simulink model "Assignment_2_1_compare_MIT_based_with_modified_MIT_based"  (R2023b)
settings: Solver=ode45  StartTime=0.0  StopTime=100  MaxStep=2.0  RelTol=1e-3
libraries: dspfdesign x4
settings Model: Creator=User  LastModifiedBy=User

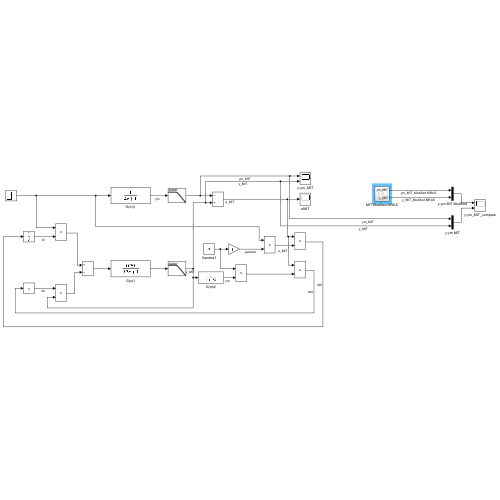
[thumbnail: Simulink's stored preview of the top-level diagram]
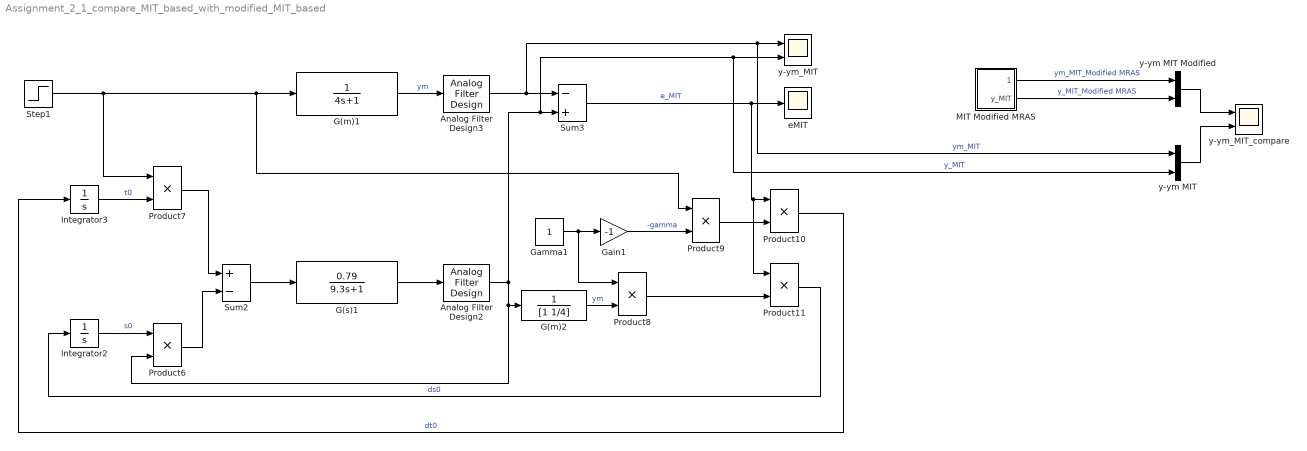
== system Assignment_2_1_compare_MIT_based_with_modified_MIT_based ==
  Analog Filter Design2 : dspfdesign/Analog Filter Design  method=Butterworth  filttype=Lowpass  N=4  Wlo=30  Whi=80  Rp=2  Rs=40
  Analog Filter Design3 : dspfdesign/Analog Filter Design  method=Butterworth  filttype=Lowpass  N=4  Wlo=30  Whi=80  Rp=2  Rs=40
  G(m)1 : TransferFcn  Denominator=[4 1]
  G(m)2 : TransferFcn  Denominator=[1 1/4]
  G(s)1 : TransferFcn  Numerator=[0.79]  Denominator=[9.3 1]
  Gain1 : Gain  Gain=-1
  Gamma1 : Constant
  Integrator2 : Integrator
  Integrator3 : Integrator
  MIT Modified MRAS : Subsystem
  Product{6..11} (6 alike) : Product
  Step1 : Step  Time=0  SampleTime=0
  Sum2 : Sum  Inputs=+-
  Sum3 : Sum  Inputs=-+
  eMIT : Scope
  y-ym MIT : Mux  Inputs=2
  y-ym MIT Modified : Mux  Inputs=2
  y-ym_MIT : Scope  NumInputPorts=2
  y-ym_MIT_compare : Scope  NumInputPorts=2
  wires:
  Integrator2/1 -> Product6/1  "s0"
  Product8/1 -> Product11/2
  Product7/1 -> Sum2/1
  Product9/1 -> Product10/2
  Sum3/1 -> Product11/1, Product10/1, eMIT/1  "e_MIT"
  Product11/1 -> Integrator2/1  "ds0"
  Integrator3/1 -> Product7/2  "t0"
  Gain1/1 -> Product9/2  "-gamma"
  Product10/1 -> Integrator3/1  "dt0"
  Gamma1/1 -> Product8/1, Gain1/1
  G(m)1/1 -> Analog Filter Design3/1  "ym"
  Step1/1 -> Product9/1, G(m)1/1, Product7/1
  G(s)1/1 -> Analog Filter Design2/1
  Analog Filter Design3/1 -> y-ym MIT/1, y-ym_MIT/1, Sum3/1  "ym_MIT"
  Analog Filter Design2/1 -> G(m)2/1, Product6/2, y-ym MIT/2, y-ym_MIT/2, Sum3/2  "y_MIT"
  Product6/1 -> Sum2/2
  Sum2/1 -> G(s)1/1
  G(m)2/1 -> Product8/2  "ym"
  y-ym MIT/1 -> y-ym_MIT_compare/2
  y-ym MIT Modified/1 -> y-ym_MIT_compare/1
  MIT Modified MRAS/1(ym_MIT) -> y-ym MIT Modified/1  "ym_MIT_Modified MRAS"
  MIT Modified MRAS/2(y_MIT) -> y-ym MIT Modified/2  "y_MIT_Modified MRAS"

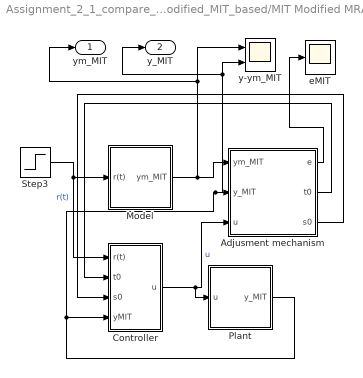
== system Assignment_2_1_compare_MIT_based_with_modified_MIT_based/MIT Modified MRAS ==
  Adjusment mechanism : Subsystem
  Controller : Subsystem
  Model : Subsystem
  Plant : Subsystem
  Step3 : Step  Time=0  SampleTime=0
  eMIT : Scope
  y-ym_MIT : Scope  NumInputPorts=2
  ym_MIT : Outport
  y_MIT : Outport  Port=2
  wires:
  Step3/1 -> Controller/1(r(t)), Model/1(r(t))  "r(t)"
  Adjusment mechanism/2(t0) -> Controller/2(t0)
  Plant/1(y_MIT) -> y-ym_MIT/2, y_MIT/1, Adjusment mechanism/2(y_MIT), Controller/4(yMIT)
  Controller/1(u) -> Plant/1(u), Adjusment mechanism/3(u)  "u"
  Adjusment mechanism/3(s0) -> Controller/3(s0)
  Adjusment mechanism/1(e) -> eMIT/1
  Model/1(ym_MIT) -> y-ym_MIT/1, ym_MIT/1, Adjusment mechanism/1(ym_MIT)

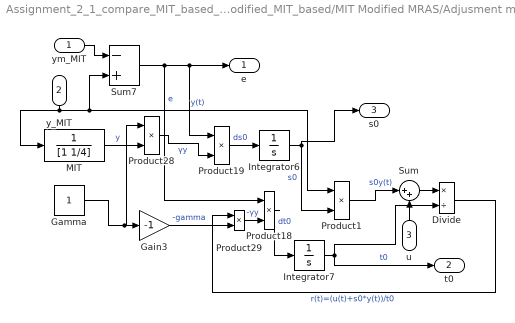
== system Assignment_2_1_compare_MIT_based_with_modified_MIT_based/MIT Modified MRAS/Adjusment mechanism ==
  ym_MIT : Inport
  y_MIT : Inport  Port=2
  u : Inport  Port=3
  Divide : Product  Inputs=*/
  Gain3 : Gain  Gain=-1
  Gamma : Constant
  Integrator6 : Integrator
  Integrator7 : Integrator  InitialCondition=0.000000000000000000000000000000000000000000000001
  MIT : TransferFcn  Denominator=[1 1/4]
  Product{1,18..19,28..29} (5 alike) : Product
  Sum : Sum  Inputs=|++
  Sum7 : Sum  Inputs=-+
  e : Outport
  t0 : Outport  Port=2
  s0 : Outport  Port=3
  wires:
  Product18/1 -> Integrator7/1  "dt0"
  y_MIT/1 -> MIT/1, Product1/1, Sum7/2  "y(t)"
  MIT/1 -> Product28/2  "y"
  Gamma/1 -> Gain3/1, Product28/1
  Product19/1 -> Integrator6/1  "ds0"
  ym_MIT/1 -> Sum7/1
  Gain3/1 -> Product29/2  "-gamma"
  Product28/1 -> Product19/2  "γy"
  Sum7/1 -> Product19/1, e/1, Product18/1  "e"
  Product29/1 -> Product18/2  "-γy"
  Integrator6/1 -> s0/1, Product1/2  "s0"
  Integrator7/1 -> Divide/2, t0/1  "t0"
  Sum/1 -> Divide/1
  Divide/1 -> Product29/1  "r(t)=(u(t)+s0*y(t))/t0"
  Product1/1 -> Sum/1  "s0y(t)"
  u/1 -> Sum/2

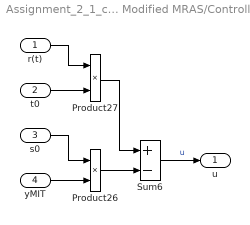
== system Assignment_2_1_compare_MIT_based_with_modified_MIT_based/MIT Modified MRAS/Controller ==
  r(t) : Inport
  t0 : Inport  Port=2
  s0 : Inport  Port=3
  yMIT : Inport  Port=4
  Product26 : Product
  Product27 : Product
  Sum6 : Sum  Inputs=+-
  u : Outport
  wires:
  Product26/1 -> Sum6/2
  r(t)/1 -> Product27/1
  Sum6/1 -> u/1  "u"
  t0/1 -> Product27/2
  s0/1 -> Product26/1
  yMIT/1 -> Product26/2
  Product27/1 -> Sum6/1

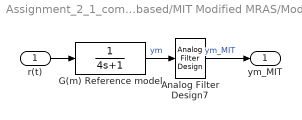
== system Assignment_2_1_compare_MIT_based_with_modified_MIT_based/MIT Modified MRAS/Model ==
  r(t) : Inport
  Analog Filter Design7 : dspfdesign/Analog Filter Design  method=Butterworth  filttype=Lowpass  N=4  Wlo=30  Whi=80  Rp=2  Rs=40
  G(m) Reference model : TransferFcn  Denominator=[4 1]
  ym_MIT : Outport
  wires:
  Analog Filter Design7/1 -> ym_MIT/1  "ym_MIT"
  G(m) Reference model/1 -> Analog Filter Design7/1  "ym"
  r(t)/1 -> G(m) Reference model/1

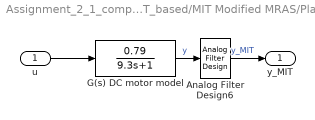
== system Assignment_2_1_compare_MIT_based_with_modified_MIT_based/MIT Modified MRAS/Plant ==
  u : Inport
  Analog Filter Design6 : dspfdesign/Analog Filter Design  method=Butterworth  filttype=Lowpass  N=4  Wlo=30  Whi=80  Rp=2  Rs=40
  G(s) DC motor model : TransferFcn  Numerator=[0.79]  Denominator=[9.3 1]
  y_MIT : Outport
  wires:
  Analog Filter Design6/1 -> y_MIT/1  "y_MIT"
  G(s) DC motor model/1 -> Analog Filter Design6/1  "y"
  u/1 -> G(s) DC motor model/1
